simulink model "motormodel"  (R2019b)
settings: Solver=VariableStepAuto  StartTime=0.0  StopTime=10.0  RelTol=1e-3
values from neighbouring files (symbols this model uses):
  A_motor = double([-bm/Jm kt/Jm 0; -kt/Lm -Rm/Lm 0; 0 0 1])    [params.m]
  B_motor = double([0; 1/Lm; 0])    [params.m]
  C_motor = eye(3)    [params.m]
settings Model: Creator=samue  LastModifiedBy=samue

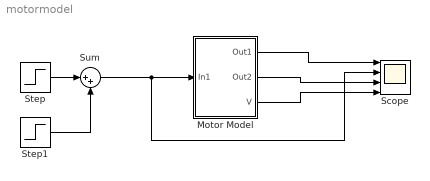
== system motormodel ==
  "Motor Model " : Subsystem
  Scope : Scope  NumInputPorts=4
  Step : Step  SampleTime=0
  Step1 : Step  Time=4  After=-1  SampleTime=0
  Sum : Sum  Inputs=|++
  wires:
  "Motor Model "/1(Out1) -> Scope/1
  Sum/1 -> "Motor Model "/1(In1), Scope/2
  Step1/1 -> Sum/2
  Step/1 -> Sum/1
  "Motor Model "/2(Out2) -> Scope/3
  "Motor Model "/3(V) -> Scope/4

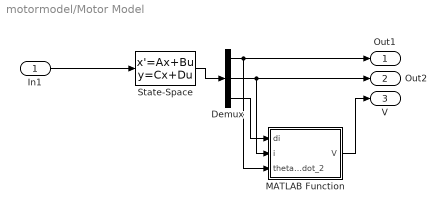
== system motormodel/Motor Model  ==
  In1 : Inport
  Demux : Demux  Outputs=3
  MATLAB Function : MATLAB Function  TreatAsAtomicUnit=on
  State-Space : StateSpace  A=A_motor  B=B_motor  C=C_motor  D=[0; 0;0]  InitialCondition=0  ContinuousStateAttributes="\"vel\""
  Out1 : Outport
  Out2 : Outport  Port=2
  V : Outport  Port=3
  wires:
  In1/1 -> State-Space/1
  State-Space/1 -> Demux/1
  Demux/1 -> Out1/1, MATLAB Function/3(theta_dot_2)
  Demux/2 -> MATLAB Function/2(i), Out2/1
  Demux/3 -> MATLAB Function/1(di)
  MATLAB Function/1(V) -> V/1

== matlab function motormodel/Motor Model /MATLAB Function ==
  data: di input; V output; i input; theta_dot_2 input
function V = fcn(di, i, theta_dot_2)
Jm = (ID + IC);
bm = 0;
Rm = 0.3;
Lm = 0.0824E-3;
kt = 7580*2*pi/60/12;
V = di*Lm + Rm*i - kt*theta_dot_2;
